simulink model "sv"  (Simulink 7.5)
settings: Solver=ode45  StartTime=0.0  StopTime=0.001  RelTol=1e-3
libraries: powerlib x16, simulink x2
settings Model: Creator=dell  LastModifiedBy=dell

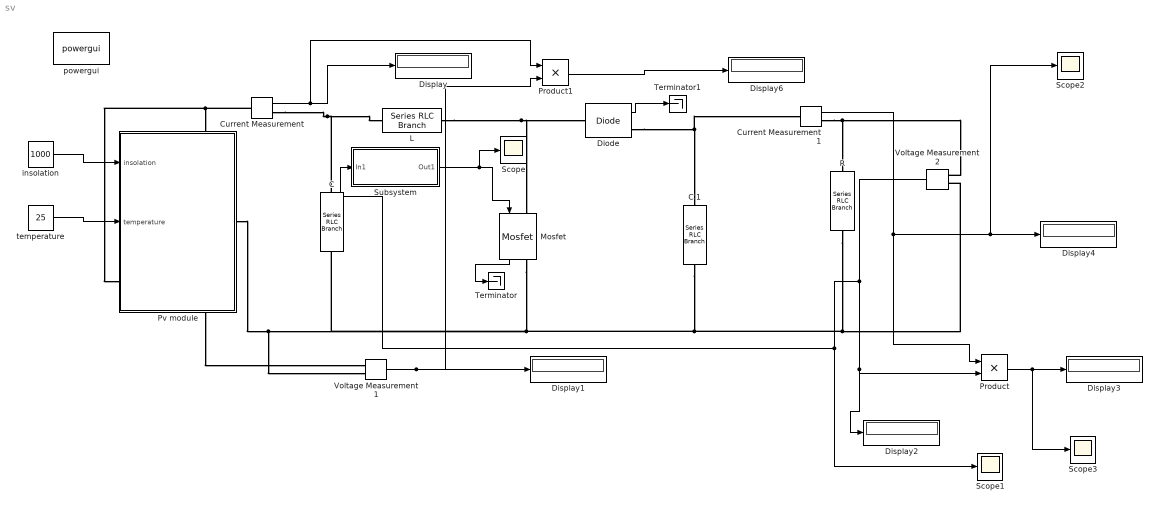
== system sv ==
  " R" : powerlib/Elements/Series RLC Branch  DialogController=POWERSYS.PowerSysDialog  PhysicalDomain=powersysdomain  SubClassName=unknown  LeftPortType=p1  RightPortType=p1  LConnTagsString=__new0  RConnTagsString=__new0  BranchType=R  Resistance=50  Inductance=1e-3  SetiL0=off  InitialCurrent=0  Capacitance=1e-6  Setx0=off  InitialVoltage=0  Measurements=None
  "C " : powerlib/Elements/Series RLC Branch  DialogController=POWERSYS.PowerSysDialog  PhysicalDomain=powersysdomain  SubClassName=unknown  LeftPortType=p1  RightPortType=p1  LConnTagsString=__new0  RConnTagsString=__new0  BranchType=C  Resistance=1  Inductance=1e-3  SetiL0=off  InitialCurrent=0  Capacitance=0.611*10^-6  Setx0=off  InitialVoltage=0  Measurements=None
  C 1 : powerlib/Elements/Series RLC Branch  DialogController=POWERSYS.PowerSysDialog  PhysicalDomain=powersysdomain  SubClassName=unknown  LeftPortType=p1  RightPortType=p1  LConnTagsString=__new0  RConnTagsString=__new0  BranchType=C  Resistance=1  Inductance=1e-3  SetiL0=off  InitialCurrent=0  Capacitance=0.611*10^-6  Setx0=off  InitialVoltage=0  Measurements=None
  Current Measurement : powerlib/Measurements/Current Measurement  DialogController=POWERSYS.PowerSysDialog  SystemSampleTime=-1  PhasorSimulation=off  OutputType=Complex  PSBequivalent=0
  Current Measurement1 : powerlib/Measurements/Current Measurement  DialogController=POWERSYS.PowerSysDialog  SystemSampleTime=-1  PhasorSimulation=off  OutputType=Complex  PSBequivalent=0
  Diode : powerlib/Power Electronics/Diode  DialogController=POWERSYS.PowerSysDialog  SystemSampleTime=-1  Ron=0.001  Lon=0  Vf=0.8  IC=0  UseSnubber=off  Rs=500  Cs=250e-9  Measurements=on
  Display{,1..4,6} (6 alike) : Display
  L : powerlib/Elements/Series RLC Branch  DialogController=POWERSYS.PowerSysDialog  PhysicalDomain=powersysdomain  SubClassName=unknown  LeftPortType=p1  RightPortType=p1  LConnTagsString=__new0  RConnTagsString=__new0  BranchType=L  Resistance=1  Inductance=7.63*10^-4  SetiL0=off  InitialCurrent=0  Capacitance=1e-6  Setx0=off  InitialVoltage=0  Measurements=None
  Mosfet : powerlib/Power Electronics/Mosfet  DialogController=POWERSYS.PowerSysDialog  SystemSampleTime=-1  Ron=0.1  Lon=0  Rd=0.01  Vfd=0  IC=0  Rs=1e5  Cs=inf  Measurements=on
  Product : Product  OutDataType=fixdt(1, 16)  OutScaling=2^0  RndMeth=Zero
  Product1 : Product  OutDataType=fixdt(1, 16)  OutScaling=2^0  RndMeth=Zero
  Pv module : Subsystem
  Scope{,1..3} (4 alike) : Scope
      Scope settings: YMin=-0.525  YMax=-0.475
      Scope1 settings: YMin=0.475  YMax=0.525
      Scope2 settings: TimeRange=0.001  YMin=0.00062  YMax=0.0007699999999999999  SaveName=ScopeData3
      Scope3 settings: TimeRange=0.001  YMin=0.00062  YMax=0.0007699999999999999  SaveName=ScopeData4
  Subsystem : Subsystem
  Terminator : Terminator
  Terminator1 : Terminator
  Voltage Measurement1 : powerlib/Measurements/Voltage Measurement  DialogController=POWERSYS.PowerSysDialog  SystemSampleTime=-1  PhasorSimulation=off  OutputType=Complex  PSBequivalent=0
  Voltage Measurement2 : powerlib/Measurements/Voltage Measurement  DialogController=POWERSYS.PowerSysDialog  SystemSampleTime=-1  PhasorSimulation=off  OutputType=Complex  PSBequivalent=0
  insolation : Constant  Value=1000  OutDataType=fixdt(1, 16)  OutScaling=2^0
  powergui : powerlib/powergui  Priority=1  SystemSampleTime=-1  SimulationMode=Continuous  SampleTime=50e-6  frequency=60  SPID=off  DisableSnubberDevices=off  DisableRonSwitches=off  DisableVfSwitches=off  SwTol=0  Interpol=off  frequencyindice=0  echomessages=off  HookPort=off  DisplayEquations=off  FunctionMessages=off  EnableUseOfTLC=off  x0status=blocks  RestoreLinks=warning  ResistiveCurrentMeasurement=off  Ylog=off  Xlog=on  ShowGrid=off  save=off  variable=ZData  ZoomFFT=off  StartTime=0.0  cycles=1  DisplayStyle=1  FreqAxis=off  MaxFrequency=1000  frequencyindicesteady=1  display=off  methode=off
  temperature : Constant  Value=25  OutDataType=fixdt(1, 16)  OutScaling=2^0  SampleTime=-1
  wires:
  insolation/1 -> Pv module/1(insolation)
  temperature/1 -> Pv module/2(temperature)
  Current Measurement/1 -> Display/1, Product1/1
  Mosfet/1 -> Terminator/1
  Voltage Measurement1/1 -> Product1/2, Display1/1
  Diode/1 -> Terminator1/1
  Voltage Measurement2/1 -> Display2/1, Product/2, Scope1/1, Subsystem/1(In1)
  Product/1 -> Display3/1, Scope3/1
  Current Measurement1/1 -> Product/1, Display4/1, Scope2/1
  Product1/1 -> Display6/1
  Subsystem/1(Out1) -> Mosfet/1, Scope/1
  connections:
  Current Measurement/LConn1 -- Pv module/LConn1 -- Voltage Measurement1/LConn1
  "C "/LConn1 -- Current Measurement/RConn1 -- L/LConn1
  " R"/RConn1 -- C 1/RConn1 -- Mosfet/RConn1 -- "C "/RConn1 -- Pv module/RConn1 -- Voltage Measurement1/LConn2 -- Voltage Measurement2/LConn2
  L/RConn1 -- Diode/LConn1 -- Mosfet/LConn1
  Diode/RConn1 -- C 1/LConn1 -- Current Measurement1/LConn1
  Current Measurement1/RConn1 -- " R"/LConn1 -- Voltage Measurement2/LConn1

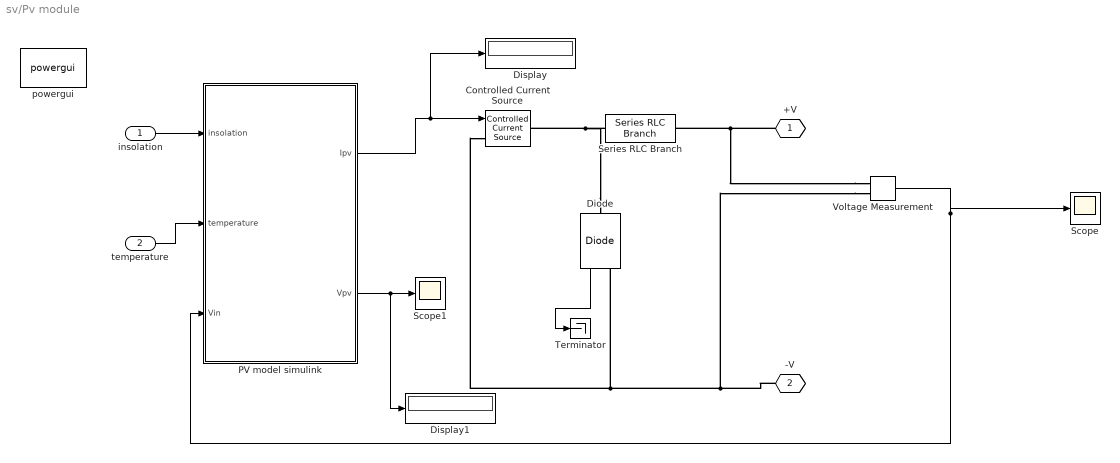
== system sv/Pv module ==
  insolation : Inport  OutDataType=fixdt(1, 16)  OutScaling=2^0
  temperature : Inport  Port=2  OutDataType=fixdt(1, 16)  OutScaling=2^0
  Controlled Current Source : powerlib/Electrical Sources/Controlled Current Source  DialogController=POWERSYS.PowerSysDialog  SystemSampleTime=-1  Initialize=on  Source_Type=DC  Amplitude=0  Phase=0  Frequency=0  Measurements=None
  Diode : powerlib/Power Electronics/Diode  DialogController=POWERSYS.PowerSysDialog  SystemSampleTime=-1  Ron=0.001  Lon=0  Vf=25  IC=0  UseSnubber=off  Rs=0  Cs=0  Measurements=on
  Display : Display
  Display1 : Display
  PV model simulink : Subsystem
  Scope : Scope
      settings: YMin=18.9973  YMax=19.0025  SaveName=ScopeData5
  Scope1 : Scope
      settings: SaveName=ScopeData6
  Series RLC Branch : powerlib/Elements/Series RLC Branch  DialogController=POWERSYS.PowerSysDialog  PhysicalDomain=powersysdomain  SubClassName=unknown  LeftPortType=p1  RightPortType=p1  LConnTagsString=__new0  RConnTagsString=__new0  BranchType=R  Resistance=0.001  Inductance=1e-3  SetiL0=off  InitialCurrent=0  Capacitance=1e-6  Setx0=off  InitialVoltage=0  Measurements=None
  Terminator : Terminator
  Voltage Measurement : powerlib/Measurements/Voltage Measurement  DialogController=POWERSYS.PowerSysDialog  SystemSampleTime=-1  PhasorSimulation=off  OutputType=Complex  PSBequivalent=0
  powergui : powerlib/powergui  Priority=1  SystemSampleTime=-1  SimulationMode=Continuous  SampleTime=50e-6  frequency=60  SPID=off  DisableSnubberDevices=off  DisableRonSwitches=off  DisableVfSwitches=off  SwTol=0  Interpol=off  frequencyindice=60  echomessages=off  HookPort=off  DisplayEquations=off  FunctionMessages=off  EnableUseOfTLC=off  x0status=blocks  RestoreLinks=warning  ResistiveCurrentMeasurement=off  Ylog=off  Xlog=on  ShowGrid=off  save=off  variable=ZData  ZoomFFT=off  StartTime=0.0  cycles=1  DisplayStyle=1  FreqAxis=off  MaxFrequency=1000  frequencyindicesteady=1  display=off  methode=off
  +V : PMIOPort  Tag=PMCPort  Port=1  Side=Left
  -V : PMIOPort  Tag=PMCPort  Port=2  Side=Right
  wires:
  PV model simulink/1(Ipv) -> Controlled Current Source/1, Display/1
  insolation/1 -> PV model simulink/1(insolation)
  Diode/1 -> Terminator/1
  PV model simulink/2(Vpv) -> Scope1/1, Display1/1
  temperature/1 -> PV model simulink/2(temperature)
  Voltage Measurement/1 -> PV model simulink/3(Vin), Scope/1
  connections:
  Diode/LConn1 -- Series RLC Branch/LConn1 -- Controlled Current Source/RConn1
  Voltage Measurement/LConn1 -- +V/RConn1 -- Series RLC Branch/RConn1
  Voltage Measurement/LConn2 -- -V/RConn1 -- Diode/RConn1 -- Controlled Current Source/LConn1

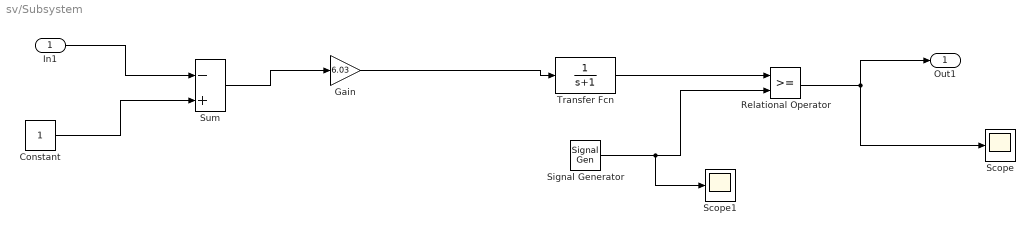
== system sv/Subsystem ==
  In1 : Inport  OutDataType=fixdt(1, 16)  OutScaling=2^0
  Constant : Constant  OutDataType=fixdt(1, 16)  OutScaling=2^0
  Gain : Gain  Gain=6.03  ParameterDataType=fixdt(1, 16)  ParameterScaling=2^0  OutDataType=fixdt(1, 16)  OutScaling=2^0
  Relational Operator : RelationalOperator  LogicOutDataTypeMode=boolean  LogicDataType=fixdt(0, 8)  OutDataTypeStr=boolean
  Scope : Scope
      settings: SaveName=ScopeData2
  Scope1 : Scope
      settings: TickLabels=on  TimeRange=0.001
  Signal Generator : SignalGenerator  WaveForm=sawtooth  Amplitude=20  Frequency=100000
  Sum : Sum  Inputs=|-+  OutDataType=fixdt(1, 16)  OutScaling=2^0
  Transfer Fcn : TransferFcn  Denominator=[1 1]
  Out1 : Outport  OutDataType=fixdt(1, 16)  OutScaling=2^0
  wires:
  In1/1 -> Sum/1
  Constant/1 -> Sum/2
  Sum/1 -> Gain/1
  Gain/1 -> Transfer Fcn/1
  Transfer Fcn/1 -> Relational Operator/1
  Signal Generator/1 -> Relational Operator/2, Scope1/1
  Relational Operator/1 -> Out1/1, Scope/1

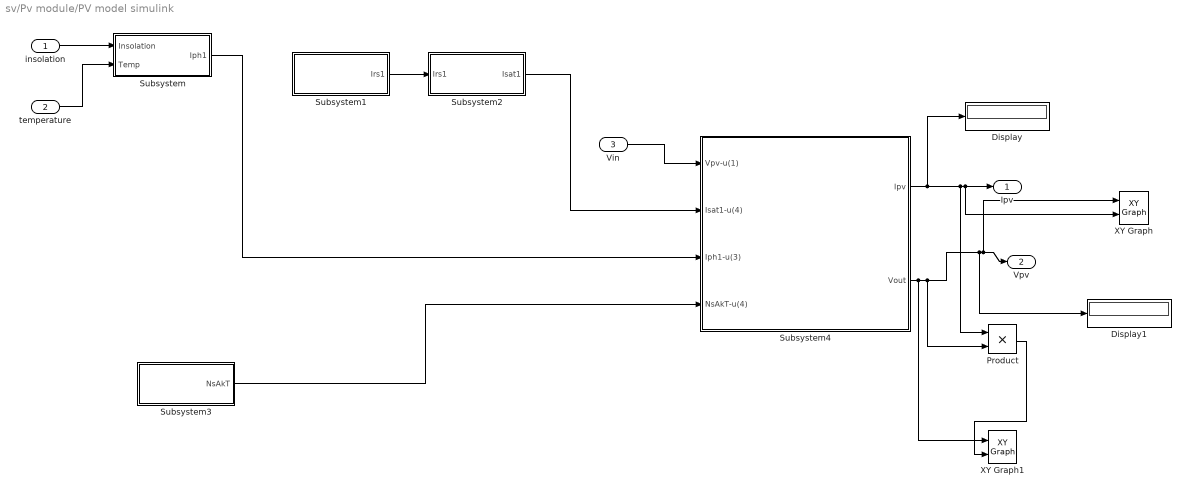
== system sv/Pv module/PV model simulink ==
  insolation : Inport  OutDataType=fixdt(1, 16)  OutScaling=2^0
  temperature : Inport  Port=2  OutDataType=fixdt(1, 16)  OutScaling=2^0
  Vin : Inport  Port=3  OutDataType=fixdt(1, 16)  OutScaling=2^0
  Display : Display
  Display1 : Display
  Product : Product  OutDataType=fixdt(1, 16)  OutScaling=2^0  RndMeth=Zero
  Subsystem : Subsystem
  Subsystem1 : Subsystem
  Subsystem2 : Subsystem
  Subsystem3 : Subsystem
  Subsystem4 : Subsystem
  XY Graph : simulink/Sinks/XY Graph  SystemSampleTime=-1  xmin=0  xmax=25  ymin=0  ymax=4  st=-1
  XY Graph1 : simulink/Sinks/XY Graph  SystemSampleTime=-1  xmin=0  xmax=25  ymin=0  ymax=50  st=-1
  Ipv : Outport  OutDataType=fixdt(1, 16)  OutScaling=2^0
  Vpv : Outport  Port=2  OutDataType=fixdt(1, 16)  OutScaling=2^0
  wires:
  Subsystem/1(Iph1) -> Subsystem4/3(Iph1-u(3))
  Subsystem1/1(Irs1) -> Subsystem2/1(Irs1)
  Subsystem3/1(NsAkT) -> Subsystem4/4(NsAkT-u(4))
  Subsystem2/1(Isat1) -> Subsystem4/2(Isat1-u(4))
  Vin/1 -> Subsystem4/1(Vpv-u(1))
  Subsystem4/1(Ipv) -> Display/1, Ipv/1, XY Graph/2, Product/1
  Subsystem4/2(Vout) -> Product/2, Vpv/1, XY Graph/1, Display1/1, XY Graph1/1
  temperature/1 -> Subsystem/2(Temp)
  insolation/1 -> Subsystem/1(Insolation)
  Product/1 -> XY Graph1/2

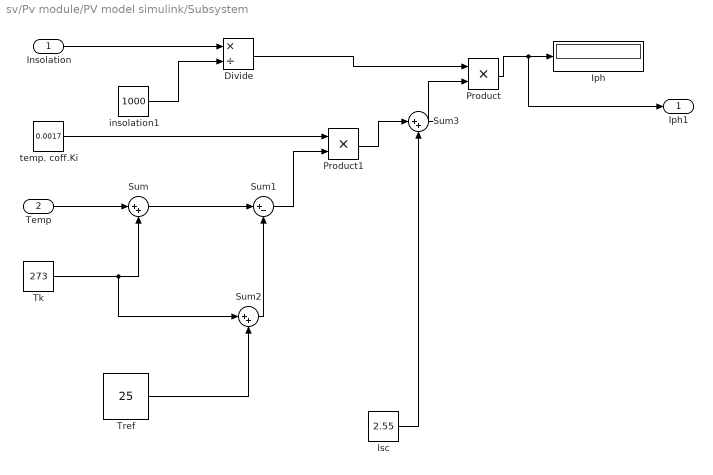
== system sv/Pv module/PV model simulink/Subsystem ==
  Insolation : Inport  OutDataType=fixdt(1, 16)  OutScaling=2^0
  Temp : Inport  Port=2  OutDataType=fixdt(1, 16)  OutScaling=2^0
  Divide : Product  Inputs=*/  OutDataType=fixdt(1, 16)  OutScaling=2^-10
  Iph : Display
  Isc : Constant  Value=2.55  OutDataType=fixdt(1, 16)  OutScaling=2^0
  Product : Product  OutDataType=fixdt(1, 16)  OutScaling=2^0  RndMeth=Zero
  Product1 : Product  OutDataType=fixdt(1, 16)  OutScaling=2^0  RndMeth=Zero
  Sum : Sum  Inputs=|++  OutDataType=fixdt(1, 16)  OutScaling=2^0
  Sum1 : Sum  Inputs=|+-  OutDataType=fixdt(1, 16)  OutScaling=2^0
  Sum2 : Sum  Inputs=|++  OutDataType=fixdt(1, 16)  OutScaling=2^0
  Sum3 : Sum  Inputs=|++  OutDataType=fixdt(1, 16)  OutScaling=2^0
  Tk : Constant  Value=273  OutDataType=fixdt(1, 16)  OutScaling=2^0
  Tref : Constant  Value=25  OutDataType=fixdt(1, 16)  OutScaling=2^0
  insolation1 : Constant  Value=1000  OutDataType=fixdt(1, 16)  OutScaling=2^0
  temp. coff.Ki : Constant  Value=0.0017  OutDataType=fixdt(1, 16)  OutScaling=2^0
  Iph1 : Outport  OutDataType=fixdt(1, 16)  OutScaling=2^0
  wires:
  Product/1 -> Iph/1, Iph1/1
  temp. coff.Ki/1 -> Product1/1
  Temp/1 -> Sum/1
  Tk/1 -> Sum/2, Sum2/1
  Sum/1 -> Sum1/1
  Tref/1 -> Sum2/2
  Sum2/1 -> Sum1/2
  Sum1/1 -> Product1/2
  Product1/1 -> Sum3/1
  Isc/1 -> Sum3/2
  Sum3/1 -> Product/2
  Insolation/1 -> Divide/1
  Divide/1 -> Product/1
  insolation1/1 -> Divide/2

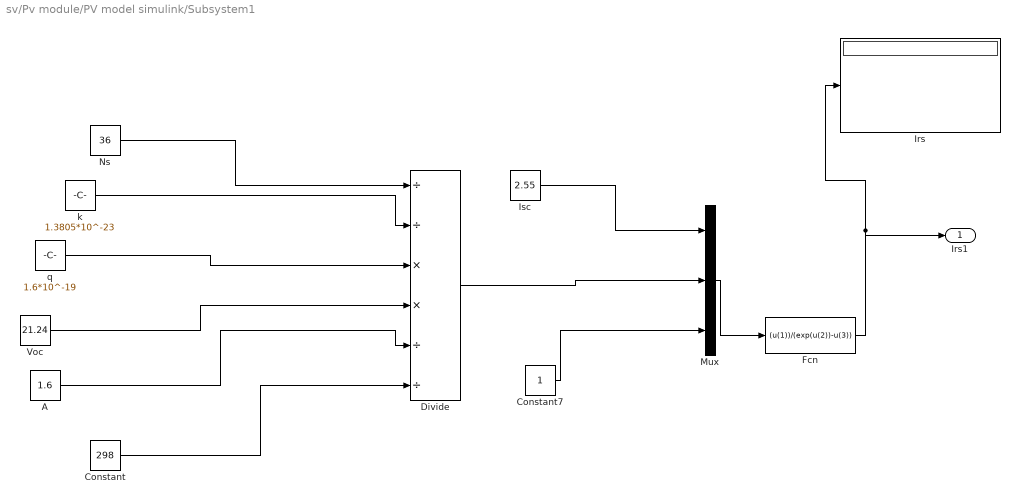
== system sv/Pv module/PV model simulink/Subsystem1 ==
  A : Constant  Value=1.6  OutDataType=fixdt(1, 16)  OutScaling=2^0
  Constant : Constant  Value=298  OutDataType=fixdt(1, 16)  OutScaling=2^0
  Constant7 : Constant  OutDataType=fixdt(1, 16)  OutScaling=2^0
  Divide : Product  Inputs=//**//  OutDataType=fixdt(1, 16)  OutScaling=2^-10
  Fcn : Fcn  Expr=(u(1))/(exp(u(2))-u(3))
  Irs : Display
      settings: Format=short_e
  Isc : Constant  Value=2.55  OutDataType=fixdt(1, 16)  OutScaling=2^0
  Mux : Mux  Inputs=3
  Ns : Constant  Value=36  OutDataType=fixdt(1, 16)  OutScaling=2^0
  Voc : Constant  Value=21.24  OutDataType=fixdt(1, 16)  OutScaling=2^0
  k : Constant  Value=1.3805*10^-23  OutDataType=fixdt(1, 16)  OutScaling=2^0
  q : Constant  Value=1.6*10^-19  OutDataType=fixdt(1, 16)  OutScaling=2^0
  Irs1 : Outport  OutDataType=fixdt(1, 16)  OutScaling=2^0
  wires:
  Ns/1 -> Divide/1
  k/1 -> Divide/2
  q/1 -> Divide/3
  Voc/1 -> Divide/4
  A/1 -> Divide/5
  Constant/1 -> Divide/6
  Isc/1 -> Mux/1
  Divide/1 -> Mux/2
  Mux/1 -> Fcn/1
  Fcn/1 -> Irs/1, Irs1/1
  Constant7/1 -> Mux/3

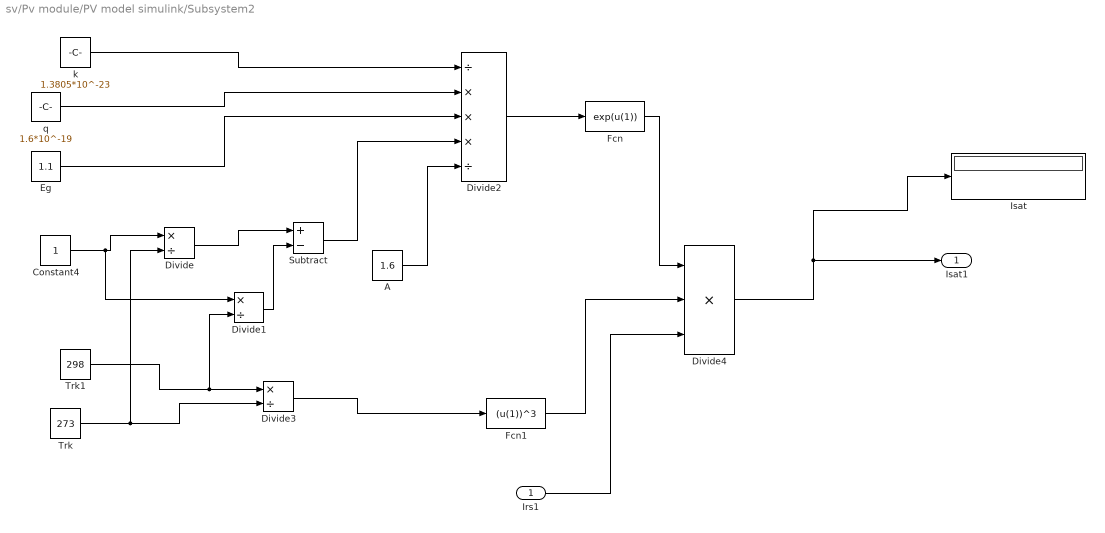
== system sv/Pv module/PV model simulink/Subsystem2 ==
  Irs1 : Inport  OutDataType=fixdt(1, 16)  OutScaling=2^0
  A : Constant  Value=1.6  OutDataType=fixdt(1, 16)  OutScaling=2^0
  Constant4 : Constant  OutDataType=fixdt(1, 16)  OutScaling=2^0
  Divide : Product  Inputs=*/  OutDataType=fixdt(1, 16)  OutScaling=2^-10
  Divide1 : Product  Inputs=*/  OutDataType=fixdt(1, 16)  OutScaling=2^-10
  Divide2 : Product  Inputs=/***/  OutDataType=fixdt(1, 16)  OutScaling=2^-10
  Divide3 : Product  Inputs=*/  OutDataType=fixdt(1, 16)  OutScaling=2^-10
  Divide4 : Product  Inputs=***  OutDataType=fixdt(1, 16)  OutScaling=2^-10
  Eg : Constant  Value=1.1  OutDataType=fixdt(1, 16)  OutScaling=2^0
  Fcn : Fcn  Expr=exp(u(1))
  Fcn1 : Fcn  Expr=(u(1))^3
  Isat : Display
  Subtract : Sum  Inputs=+-  OutDataType=fixdt(1, 16)  OutScaling=2^-10
  Trk : Constant  Value=273  OutDataType=fixdt(1, 16)  OutScaling=2^0
  Trk1 : Constant  Value=298  OutDataType=fixdt(1, 16)  OutScaling=2^0
  k : Constant  Value=1.3805*10^-23  OutDataType=fixdt(1, 16)  OutScaling=2^0
  q : Constant  Value=1.6*10^-19  OutDataType=fixdt(1, 16)  OutScaling=2^0
  Isat1 : Outport  OutDataType=fixdt(1, 16)  OutScaling=2^0
  wires:
  k/1 -> Divide2/1
  q/1 -> Divide2/2
  Eg/1 -> Divide2/3
  Constant4/1 -> Divide/1, Divide1/1
  Trk1/1 -> Divide3/1, Divide1/2
  Trk/1 -> Divide3/2, Divide/2
  Divide/1 -> Subtract/1
  Divide1/1 -> Subtract/2
  Subtract/1 -> Divide2/4
  A/1 -> Divide2/5
  Divide2/1 -> Fcn/1
  Divide4/1 -> Isat/1, Isat1/1
  Fcn/1 -> Divide4/1
  Divide3/1 -> Fcn1/1
  Fcn1/1 -> Divide4/2
  Irs1/1 -> Divide4/3

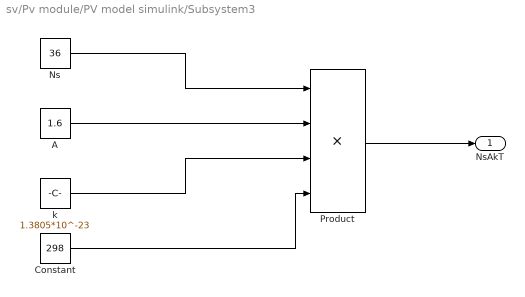
== system sv/Pv module/PV model simulink/Subsystem3 ==
  A : Constant  Value=1.6  OutDataType=fixdt(1, 16)  OutScaling=2^0
  Constant : Constant  Value=298  OutDataType=fixdt(1, 16)  OutScaling=2^0
  Ns : Constant  Value=36  OutDataType=fixdt(1, 16)  OutScaling=2^0
  Product : Product  Inputs=4  OutDataType=fixdt(1, 16)  OutScaling=2^0  RndMeth=Zero
  k : Constant  Value=1.3805*10^-23  OutDataType=fixdt(1, 16)  OutScaling=2^0
  NsAkT : Outport  OutDataType=fixdt(1, 16)  OutScaling=2^0
  wires:
  Ns/1 -> Product/1
  A/1 -> Product/2
  k/1 -> Product/3
  Constant/1 -> Product/4
  Product/1 -> NsAkT/1

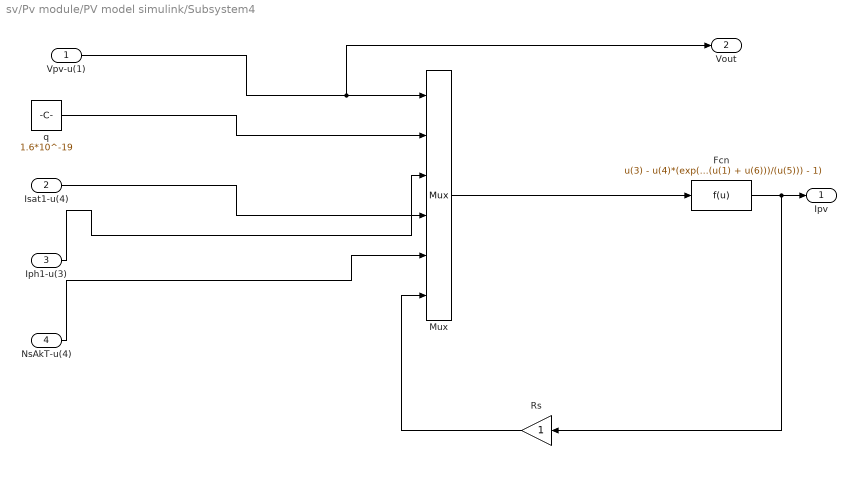
== system sv/Pv module/PV model simulink/Subsystem4 ==
  Vpv-u(1) : Inport  OutDataType=fixdt(1, 16)  OutScaling=2^0
  Isat1-u(4) : Inport  Port=2  OutDataType=fixdt(1, 16)  OutScaling=2^0
  Iph1-u(3) : Inport  Port=3  OutDataType=fixdt(1, 16)  OutScaling=2^0
  NsAkT-u(4) : Inport  Port=4  OutDataType=fixdt(1, 16)  OutScaling=2^0
  Fcn : Fcn  Expr=u(3) - u(4)*(exp((u(2)*(u(1) + u(6)))/(u(5))) - 1)
  Mux : Mux  Inputs=6
  Rs : Gain  ParameterDataType=fixdt(1, 16)  ParameterScaling=2^0  OutDataType=fixdt(1, 16)  OutScaling=2^0
  q : Constant  Value=1.6*10^-19  OutDataType=fixdt(1, 16)  OutScaling=2^0
  Ipv : Outport  OutDataType=fixdt(1, 16)  OutScaling=2^0
  Vout : Outport  Port=2  OutDataType=fixdt(1, 16)  OutScaling=2^0
  wires:
  Vpv-u(1)/1 -> Mux/1, Vout/1
  q/1 -> Mux/2
  NsAkT-u(4)/1 -> Mux/5
  Mux/1 -> Fcn/1
  Fcn/1 -> Ipv/1, Rs/1
  Isat1-u(4)/1 -> Mux/4
  Iph1-u(3)/1 -> Mux/3
  Rs/1 -> Mux/6
